simulink model "GFLIB_ControllerPIDpAW_BAM"  (Simulink 9.3)
settings: Solver=VariableStepAuto  StartTime=0.0  StopTime=10.0  RelTol=1e-3
settings Model: Creator=nxa18952  LastModifiedBy=nxa18952
settings DataIOCC: SaveFormat=Dataset  SignalLoggingSaveFormat=Dataset  ReturnWorkspaceOutputs=on
settings OptimizationCC: LifeSpan=auto
settings DebuggingCC: UnderspecifiedInitializationDetection=Simplified  MergeDetectMultiDrivingBlocksExec=error  FcnCallInpInsideContextMsg=error  SFUnexpectedBacktrackingDiag=error  SFNoUnconditionalDefaultTransitionDiag=error  SFExecutionAtInitializationDiag=warning  ArithmeticOperatorsInVariantConditions=error
settings HardwareCC: ProdBitPerPointer=64  ProdBitPerSizeT=64  ProdBitPerPtrDiffT=64  ProdLargestAtomicFloat=Float  ProdIntDivRoundTo=Zero  ProdEndianess=LittleEndian  ProdWordSize=64  ProdHWDeviceType=Intel->x86-64 (Windows64)
settings ModelReferenceCC: PropagateSignalLabelsOutOfModel=on
settings SFSimCC: SimUseLocalCustomCode=on
settings RTWCC: RTWUseLocalCustomCode=on
settings CodeAppCC: StateflowObjectComments=off
settings GRTTargetCC: TargetLangStandard=C99 (ISO)  CombineOutputUpdateFcns=on  GRTInterface=off
settings ConfigComp: CovMetricSettings=dwe  CovHtmlReporting=off  CovSaveCumulativeToWorkspaceVar=off  CovSaveSingleToWorkspaceVar=off  CovExternalEMLEnable=on

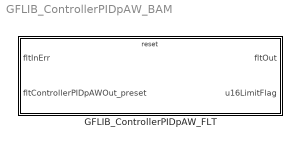
== system GFLIB_ControllerPIDpAW_BAM ==
  GFLIB_ControllerPIDpAW_FLT : Subsystem  TreatAsAtomicUnit=on  mask(GFLIB_ControllerPIDpAW_FLT){showStates=Hide (faster execution), resetStatesEnable=Pre-set according to the first set of inputs after reset, fltPropGain=0, fltIntegGain=0, fltDerivGain=0, fltFiltCoef=0, fltLowerLimit=0, fltUpperLimit=0}
      mask prompts: showStates "Show internal states"; resetStatesEnable "Internal state after reset"; fltPropGain "fltPropGain (Proportional gain)"; fltIntegGain "fltIntegGain (Integral gain)"; fltDerivGain "fltDerivGain (Derivative Gain)"; fltFiltCoef "fltFiltCoef (Derivative term filter coefficient)"; fltLowerLimit "fltLowerLimit (Lower Limit of the controller)"; fltUpperLimit "fltUpperLimit (Upper Limit of the controller)"
      mask help: Parallel form PID controller with anti-windup in single precision floating-point implementation. This block supports re-initialization of the internal state during simulation. If the block is reset, the controller's output will be aligned with the input fltControllerPIDpAWOut_preset. Refer to the AMMCLIB User's Guide for further details.
      mask init:
      | if ~evalin('base','exist(''tS8'',''var'')')
      |   if (2 ~= exist('SWLIBS_Typedefs.mat','file'))
      |       error('File SWLIBS_Typedefs.mat is not on the Matlab path. Please add the AMMCLIB "bam" folder in the Matlab Search Path.');
      |   else
      |       evalin('base', 'load(''SWLIBS_Typedefs.mat'')');
      |   end
      | end
      | if showStates == 1
      |     % hidden state variables
      |     if strcmp(get_param([gcb '/fltPropGain'], 'BlockType'), 'Inport')
      |         posblk = get_param(gcb, 'Position');
      | 
      |         pos = get_param(    [gcb, '/fltPropGain'], 'Position');
      |         orient = get_param( [gcb, '/fltPropGain'], 'Orientation');
      |         delete_block(       [gcb, '/fltPropGain']);
      |         add_block('built-in/Ground', [gcb, '/fltPropGain'], 'Position', pos, 'Orientation', orient);
      | 
      |         pos = get_param(    [gcb, '/fltIntegGain'], 'Position');
      |         orient = get_param( [gcb, '/fltIntegGain'], 'Orientation');
      |         delete_block(       [gcb, '/fltIntegGain']);
      |         add_block('built-in/Ground', [gcb, '/fltIntegGain'], 'Position', pos, 'Orientation', orient);
      | 
      |         pos = get_param(    [gcb, '/fltDerivGain'], 'Position');
      |         orient = get_param( [gcb, '/fltDerivGain'], 'Orientation');
      |         delete_block(       [gcb, '/fltDerivGain']);
      |         add_block('built-in/Ground', [gcb, '/fltDerivGain'], 'Position', pos, 'Orientation', orient);
      | 
      |         pos = get_param(    [gcb, '/fltFiltCoef'], 'Position');
      |         orient = get_param( [gcb, '/fltFiltCoef'], 'Orientation');
      |         delete_block(       [gcb, '/fltFiltCoef']);
      |         add_block('built-in/Ground', [gcb, '/fltFiltCoef'], 'Position', pos, 'Orientation', orient);
      | 
      |         pos = get_param(    [gcb, '/fltLowerLimit'], 'Position');
      |         orient = get_param( [gcb, '/fltLowerLimit'], 'Orientation');
      |         delete_block(       [gcb, '/fltLowerLimit']);
      |         add_block('built-in/Ground', [gcb, '/fltLowerLimit'], 'Position', pos, 'Orientation', orient);
      | 
      |         pos = get_param(    [gcb, '/fltUpperLimit'], 'Position');
      |         orient = get_param( [gcb, '/fltUpperLimit'], 'Orientation');
      |         delete_block(       [gcb, '/fltUpperLimit']);
      |         add_block('built-in/Ground', [gcb, '/fltUpperLimit'], 'Position', pos, 'Orientation', orient);
      | 
      |         pos = get_param(    [gcb, '/fltIntegPartK_1'], 'Position');
      |         orient = get_param( [gcb, '/fltIntegPartK_1'], 'Orientation');
      |         delete_block(       [gcb, '/fltIntegPartK_1']);
      |         add_block('built-in/Ground', [gcb, '/fltIntegPartK_1'], 'Position', pos, 'Orientation', orient);
      | 
      |         pos = get_param(    [gcb, '/fltDerivPartK_1'], 'Position');
      |         orient = get_param( [gcb, '/fltDerivPartK_1'], 'Orientation');
      |         delete_block(       [gcb, '/fltDerivPartK_1']);
      |         add_block('built-in/Ground', [gcb, '/fltDerivPartK_1'], 'Position', pos, 'Orientation', orient);
      | 
      |         pos = get_param(    [gcb, '/fltInK_1'], 'Position');
      |         orient = get_param( [gcb, '/fltInK_1'], 'Orientation');
      |         delete_block(       [gcb, '/fltInK_1']);
      |         add_block('built-in/Ground', [gcb, '/fltInK_1'], 'Position', pos, 'Orientation', orient);
      | 
      | 
      |         pos = get_param(    [gcb '/fltIntegPartK_1_Out'], 'Position');
      |         orient = get_param( [gcb '/fltIntegPartK_1_Out'], 'Orientation');
      |         delete_block(       [gcb '/fltIntegPartK_1_Out']);
      |         add_block('built-in/Terminator', [gcb '/fltIntegPartK_1_Out'], 'Position', pos, 'Orientation', orient);
      | 
      |         pos = get_param(    [gcb '/fltDerivPartK_1_Out'], 'Position');
      |         orient = get_param( [gcb '/fltDerivPartK_1_Out'], 'Orientation');
      |         delete_block(       [gcb '/fltDerivPartK_1_Out']);
      |         add_block('built-in/Terminator', [gcb '/fltDerivPartK_1_Out'], 'Position', pos, 'Orientation', orient);
      | 
      |         pos = get_param(    [gcb '/fltInK_1_Out'], 'Position');
      |         orient = get_param( [gcb '/fltInK_1_Out'], 'Orientation');
      |         delete_block(       [gcb '/fltInK_1_Out']);
      |         add_block('built-in/Terminator', [gcb '/fltInK_1_Out'], 'Position', pos, 'Orientation', orient);
      | 
      | 
      |         set_param([gcb '/fltInErr'], 'Port', '1');
      |         set_param([gcb '/fltControllerPIDpAWOut_preset'], 'Port', '2');
      | 
      |         set_param([gcb '/fltOut'], 'Port', '1');
      |         set_param([gcb '/u16LimitFlag'], 'Port', '2');
      | 
      |         set_param(gcb,'MaskEnables',{'on','on','on','on','on','on','on','on'});
      | 
      |         if (posblk(4) - posblk(2)) > 75
      |           height = 75;
      |           set_param(gcb,'Position',[posblk(1), posblk(2), posblk(3), posblk(2)+height])
      |         end
      |     end
      | else
      |     % shown state variables
      |     if strcmp(get_param([gcb '/fltPropGain'], 'BlockType'), 'Ground')
      |         posblk = get_param(gcb, 'Position');
      | 
      |         pos = get_param(    [gcb, '/fltPropGain'], 'Position');
      |         orient = get_param( [gcb, '/fltPropGain'], 'Orientation');
      |         delete_block(       [gcb, '/fltPropGain']);
      |         add_block('built-in/Inport', [gcb, '/fltPropGain'], 'Position', pos, 'Orientation', orient, 'OutDataTypeStr', 'single');
      | 
      |         pos = get_param(    [gcb, '/fltIntegGain'], 'Position');
      |         orient = get_param( [gcb, '/fltIntegGain'], 'Orientation');
      |         delete_block(       [gcb, '/fltIntegGain']);
      |         add_block('built-in/Inport', [gcb, '/fltIntegGain'], 'Position', pos, 'Orientation', orient, 'OutDataTypeStr', 'single');
      | 
      |         pos = get_param(    [gcb, '/fltDerivGain'], 'Position');
      |         orient = get_param( [gcb, '/fltDerivGain'], 'Orientation');
      |         delete_block(       [gcb, '/fltDerivGain']);
      |         add_block('built-in/Inport', [gcb, '/fltDerivGain'], 'Position', pos, 'Orientation', orient, 'OutDataTypeStr', 'single');
      | 
      |         pos = get_param(    [gcb, '/fltFiltCoef'], 'Position');
      |         orient = get_param( [gcb, '/fltFiltCoef'], 'Orientation');
      |         delete_block(       [gcb, '/fltFiltCoef']);
      |         add_block('built-in/Inport', [gcb, '/fltFiltCoef'], 'Position', pos, 'Orientation', orient, 'OutDataTypeStr', 'single');
      | 
      |         pos = get_param(    [gcb, '/fltLowerLimit'], 'Position');
      |         orient = get_param( [gcb, '/fltLowerLimit'], 'Orientation');
      |         delete_block(       [gcb, '/fltLowerLimit']);
      |         add_block('built-in/Inport', [gcb, '/fltLowerLimit'], 'Position', pos, 'Orientation', orient, 'OutDataTypeStr', 'single');
      | 
      |         pos = get_param(    [gcb, '/fltUpperLimit'], 'Position');
      |         orient = get_param( [gcb, '/fltUpperLimit'], 'Orientation');
      |         delete_block(       [gcb, '/fltUpperLimit']);
      |         add_block('built-in/Inport', [gcb, '/fltUpperLimit'], 'Position', pos, 'Orientation', orient, 'OutDataTypeStr', 'single');
      | 
      |         pos = get_param(    [gcb, '/fltIntegPartK_1'], 'Position');
      |         orient = get_param( [gcb, '/fltIntegPartK_1'], 'Orientation');
      |         delete_block(       [gcb, '/fltIntegPartK_1']);
      |         add_block('built-in/Inport', [gcb, '/fltIntegPartK_1'], 'Position', pos, 'Orientation', orient, 'OutDataTypeStr', 'single');
      | 
      |         pos = get_param(    [gcb, '/fltDerivPartK_1'], 'Position');
      |         orient = get_param( [gcb, '/fltDerivPartK_1'], 'Orientation');
      |         delete_block(       [gcb, '/fltDerivPartK_1']);
      |         add_block('built-in/Inport', [gcb, '/fltDerivPartK_1'], 'Position', pos, 'Orientation', orient, 'OutDataTypeStr', 'single');
      | 
      |         pos = get_param(    [gcb, '/fltInK_1'], 'Position');
      |         orient = get_param( [gcb, '/fltInK_1'], 'Orientation');
      |         delete_block(       [gcb, '/fltInK_1']);
      |         add_block('built-in/Inport', [gcb, '/fltInK_1'], 'Position', pos, 'Orientation', orient, 'OutDataTypeStr', 'single');
      | 
      | 
      |         pos = get_param(    [gcb '/fltIntegPartK_1_Out'], 'Position');
      |         orient = get_param( [gcb '/fltIntegPartK_1_Out'], 'Orientation');
      |         delete_block(       [gcb '/fltIntegPartK_1_Out']);
      |         add_block('built-in/Outport', [gcb '/fltIntegPartK_1_Out'], 'Position', pos, 'Orientation', orient);
      | 
      |         pos = get_param(    [gcb '/fltDerivPartK_1_Out'], 'Position');
      |         orient = get_param( [gcb '/fltDerivPartK_1_Out'], 'Orientation');
      |         delete_block(       [gcb '/fltDerivPartK_1_Out']);
      |         add_block('built-in/Outport', [gcb '/fltDerivPartK_1_Out'], 'Position', pos, 'Orientation', orient);
      | 
      |         pos = get_param(    [gcb '/fltInK_1_Out'], 'Position');
      |         orient = get_param( [gcb '/fltInK_1_Out'], 'Orientation');
      |         delete_block(       [gcb '/fltInK_1_Out']);
      |         add_block('built-in/Outport', [gcb '/fltInK_1_Out'], 'Position', pos, 'Orientation', orient);
      | 
      | 
      |         set_param([gcb '/fltInErr'], 'Port', '1');
      |         set_param([gcb '/fltControllerPIDpAWOut_preset'], 'Port', '2');
      |         set_param([gcb '/fltPropGain'], 'Port', '3');
      |         set_param([gcb '/fltIntegGain'], 'Port', '4');
      |         set_param([gcb '/fltDerivGain'], 'Port', '5');
      |         set_param([gcb '/fltFiltCoef'], 'Port', '6');
      |         set_param([gcb '/fltLowerLimit'], 'Port', '7');
      |         set_param([gcb '/fltUpperLimit'], 'Port', '8');
      |         set_param([gcb '/fltIntegPartK_1'], 'Port', '9');
      |         set_param([gcb '/fltDerivPartK_1'], 'Port', '10');
      |         set_param([gcb '/fltInK_1'], 'Port', '11');
      | 
      |         set_param([gcb '/fltOut'], 'Port', '1');
      |         set_param([gcb '/u16LimitFlag'], 'Port', '2');
      |         set_param([gcb '/fltIntegPartK_1_Out'], 'Port', '3');
      |         set_param([gcb '/fltDerivPartK_1_Out'], 'Port', '4');
      |         set_param([gcb '/fltInK_1_Out'], 'Port', '5');
      | 
      |         set_param(gcb,'MaskEnables',{'on','on','off','off','off','off','off','off'});
      | 
      |         if (posblk(4) - posblk(2)) < 300
      |           height = 300;
      |           set_param(gcb,'Position',[posblk(1), posblk(2), posblk(3), posblk(2)+height])
      |         end
      |     end
      | end
      settings: RTWSystemCode=Inline
      mask TypeOptions showStates: Hide (faster execution) | Show (allows debugging; connect feedback loops manually)
      mask Callback showStates:
      | maskStr = get_param(gcb,'showStates');
      | if strcmp(maskStr,'Hide (faster execution)'),
      |     set_param(gcb,'MaskEnables',{'on','on','on','on','on','on','on','on'});
      | else
      |     set_param(gcb,'MaskEnables',{'on','on','off','off','off','off','off','off'});
      | end
      mask TypeOptions resetStatesEnable: Pre-set according to the first set of inputs after reset | Clear to zero
      mask Display:
      | color('black');
      | pos = get_param(gcb, 'Position');
      | width = pos(3) - pos(1);
      | height = pos(4) - pos(2);
      | tX=width/2;
      | tY=height - 25;
      | color('black');
      | text(tX,tY, 'GFLIB_ControllerPIDpAW_FLT', 'horizontalAlignment', 'center');
      | if showStates == 2
      |   color('red');
      |   text(tX,tY - 20, ['debugging mode' char(13) char(10) '(limited performance)'], 'horizontalAlignment', 'center');
      | end

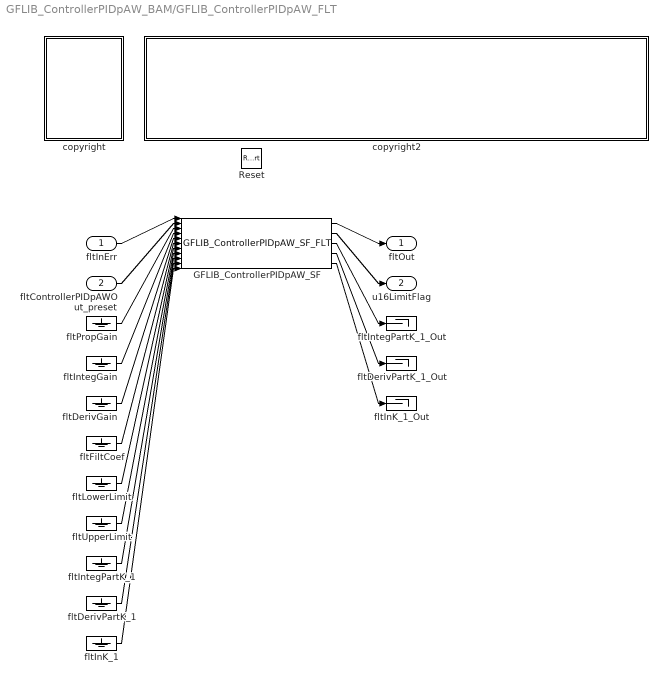
== system GFLIB_ControllerPIDpAW_BAM/GFLIB_ControllerPIDpAW_FLT ==
  fltInErr : Inport  OutDataTypeStr=single
  fltControllerPIDpAWOut_preset : Inport  Port=2  OutDataTypeStr=single
  Reset : ResetPort  DisableCoverage=on
  GFLIB_ControllerPIDpAW_SF : S-Function  FunctionName=GFLIB_ControllerPIDpAW_SF_FLT  Parameters=showStates,resetStatesEnable,fltPropGain,fltIntegGain,fltDerivGain,fltFiltCoef,fltLowerLimit,fltUpperLimit  SFunctionDeploymentMode=off  EnableBusSupport=off
  copyright : Subsystem
      mask Display: text(10,90,'FILE:');text(10,75,'DESRIPTION:');text(10,60,'COPYRIGHT:');text(10,45,'VERSION:');text(10,30,'DATE:')
  copyright2 : Subsystem
      mask Display: text(10,90,'GFLIB_ControllerPIDpAW_BAM_FLT.mdl');text(10,75,'Parallel form of a standard PID controller with anti-windup.');text(10,60,'NXP 2020');text(10,45,'1.0');text(10,30,'28-Mar-2020');
  fltDerivGain : Ground
  fltDerivPartK_1 : Ground
  fltDerivPartK_1_Out : Terminator
  fltFiltCoef : Ground
  fltInK_1 : Ground
  fltInK_1_Out : Terminator
  fltIntegGain : Ground
  fltIntegPartK_1 : Ground
  fltIntegPartK_1_Out : Terminator
  fltLowerLimit : Ground
  fltPropGain : Ground
  fltUpperLimit : Ground
  fltOut : Outport
  u16LimitFlag : Outport  Port=2
  wires:
  fltInErr/1 -> GFLIB_ControllerPIDpAW_SF/1
  fltControllerPIDpAWOut_preset/1 -> GFLIB_ControllerPIDpAW_SF/2
  fltPropGain/1 -> GFLIB_ControllerPIDpAW_SF/3
  fltIntegGain/1 -> GFLIB_ControllerPIDpAW_SF/4
  fltDerivGain/1 -> GFLIB_ControllerPIDpAW_SF/5
  fltFiltCoef/1 -> GFLIB_ControllerPIDpAW_SF/6
  fltLowerLimit/1 -> GFLIB_ControllerPIDpAW_SF/7
  fltUpperLimit/1 -> GFLIB_ControllerPIDpAW_SF/8
  fltIntegPartK_1/1 -> GFLIB_ControllerPIDpAW_SF/9
  fltDerivPartK_1/1 -> GFLIB_ControllerPIDpAW_SF/10
  fltInK_1/1 -> GFLIB_ControllerPIDpAW_SF/11
  GFLIB_ControllerPIDpAW_SF/1 -> fltOut/1
  GFLIB_ControllerPIDpAW_SF/2 -> u16LimitFlag/1
  GFLIB_ControllerPIDpAW_SF/3 -> fltIntegPartK_1_Out/1
  GFLIB_ControllerPIDpAW_SF/4 -> fltDerivPartK_1_Out/1
  GFLIB_ControllerPIDpAW_SF/5 -> fltInK_1_Out/1

== system GFLIB_ControllerPIDpAW_BAM/GFLIB_ControllerPIDpAW_FLT/copyright ==

== system GFLIB_ControllerPIDpAW_BAM/GFLIB_ControllerPIDpAW_FLT/copyright2 ==
